simulink model "VD_correct"  (R2023b)
settings: Solver=ode15s  StartTime=0.0  StopTime=10.0  RelTol=1e-3
libraries: simulink x1
settings Model: Creator=Supriya  LastModifiedBy=Supriya

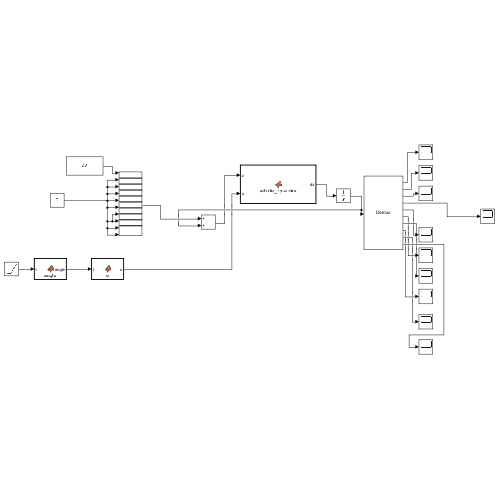
[thumbnail: Simulink's stored preview of the top-level diagram]
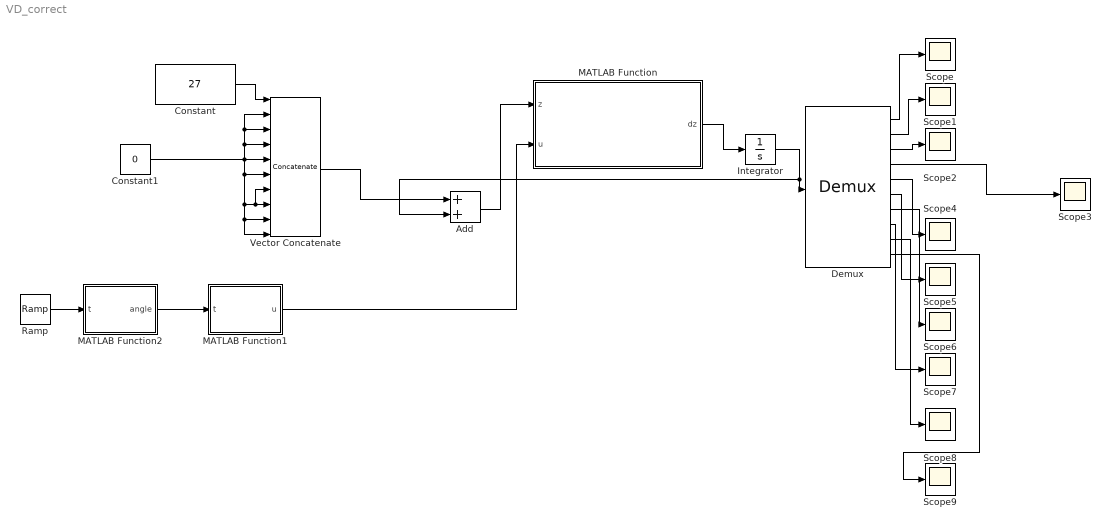
== system VD_correct ==
  Add : Sum
  Constant : Constant  Value=27
  Constant1 : Constant  Value=0
  Demux : Demux  Outputs=10
      settings: DisplayOption=none
  Integrator : Integrator
  MATLAB Function : MATLAB Function  TreatAsAtomicUnit=on
  MATLAB Function1 : MATLAB Function  TreatAsAtomicUnit=on
  MATLAB Function2 : MATLAB Function  TreatAsAtomicUnit=on
  Ramp : simulink/Sources/Ramp  slope=1  start=0  InitialOutput=0
  Scope{,1..9} (10 alike) : Scope
  Vector Concatenate : Concatenate  NumInputs=10
  wires:
  MATLAB Function/1(dz) -> Integrator/1
  Constant1/1 -> Vector Concatenate/3, Vector Concatenate/2, Vector Concatenate/4, Vector Concatenate/10, Vector Concatenate/9, Vector Concatenate/7, Vector Concatenate/8, Vector Concatenate/6, Vector Concatenate/5
  Vector Concatenate/1 -> Add/1
  Constant/1 -> Vector Concatenate/1
  Integrator/1 -> Demux/1, Add/2
  Demux/1 -> Scope/1
  Demux/2 -> Scope1/1
  Demux/3 -> Scope2/1
  Demux/4 -> Scope3/1
  Demux/5 -> Scope4/1
  Demux/6 -> Scope5/1
  Demux/7 -> Scope6/1
  Demux/8 -> Scope7/1
  MATLAB Function2/1(angle) -> MATLAB Function1/1(t)
  MATLAB Function1/1(u) -> MATLAB Function/2(u)
  Ramp/1 -> MATLAB Function2/1(t)
  Add/1 -> MATLAB Function/1(z)
  Demux/9 -> Scope8/1
  Demux/10 -> Scope9/1

== matlab function VD_correct/MATLAB Function1 ==
  data: t input; u output
function u = u(t)
    u=[1; 0; angle(t);];
end

== matlab function VD_correct/MATLAB Function ==
  data: dz output; z input; u input
function dz = vehicle_dynamics(z, u)
    % abc = Forces
    % dt;
    %tic;    
    accel = u(1);
    deccel = u(2);
    delta = u(3);
    function params = system_parameters();
        params.m = 2000; %kg
        params.rho = 1.225; %kg /m3
        params.C_d = 0.4; %
        params.Af = 1.6; %frontal area of vehicle 
        params.V_wind = 10 ;  %m/s
        params.a = 1.1;         %front_axel - CG
        params.b = 1.2;         % rear axel - CG
        params.l =  1.1 + 1.2;  %%m length of wheel base
        params.tf =  1.58; % track idth of wheel base 
        params.tr = 1.58; % track width of rear wheel base
        params.w = 1.58; % vehicle width
        params.Izz_v = 2000 * ((1.1+1.2)^2 + (1.58)^2) / 12;  %vehicle intertia 
        params.max_torque = 450; %Nm
        params.max_power =  225* 10^3;
        params.C_x = 50000 ;     %N
        params.C_y = 40000 ;  %N/Radlateral coefficient of stiffness
        params.R_f = 0.334; % m 
        params.R_r = 0.334; % m
        params.tire_m_f = 12; %mass in Kg
        params.tire_m_r = 12; %mass in Kg
        params.Iyy_w_f = 0.5 * 12 * 0.334; 
        params.Iyy_w_r = 0.5 * 12 * 0.334;
        % params.slip_max = (params.max_torque * accel / (params.R_f *2 * params.C_x));
        params.slip_min = -0.1;
        params.no_drive_wheels = 2;
        params.g = 9.8; %m/s2
        params.h = 0.25; %m
    end
    function slip_angles =  calculate_slip_angles(params,z, delta);


        Vx = z(1);
        Vy = z(2);
        r =  z(3);
        
        % term_a = atan2( (Vy + params.a * r ), ( Vx - (r * params.tf /2)) );
        % term_b = atan2( (Vy + params.a * r ), ( Vx + (r * params.tf /2)) );
        % term_c = atan2( (Vy - params.b * r ), ( Vx - (r * params.tr /2)) );
        % term_d = atan2( (Vy - params.b * r ), ( Vx + (r * params.tf /2)) );
    
        term_a = atan2( (Vy + params.a * r ),  Vx  );
        term_b = atan2( (Vy + params.a * r ),  Vx );
        term_c = atan2( (Vy - params.b * r ),  Vx );
        term_d = atan2( (Vy - params.b * r ),  Vx  );
    
        alpha_fl =  delta - term_a; if isnan(term_a ), alpha_fl = 0; end 
        alpha_fr =  delta - term_b; if isnan(term_b), alpha_fr = 0; end 
        alpha_rl = -term_c; if isnan(term_c), alpha_rl = 0; end
        alpha_rr = -term_d; if isnan(term_d), alpha_rr = 0; end
        
        slip_angles = -1 * [alpha_fl ; alpha_fr; alpha_rl; alpha_rr ];

    end
    params = system_parameters();
    function slips = caculate_slip(params, z ,deccel)
        %wheel longitudinal velocity and angular rate
        Vx = z(1);
        r = z(3);
        %%calculate linear velocities of each wheel 
           V_fl = Vx - (r * params.tf /2);
           V_fr = Vx + (r * params.tf /2);
           V_rl = Vx - (r * params.tr /2);
           V_rr = Vx + (r * params.tr /2);
           w_fl = z(7);
           w_fr = z(8);
           w_rl = z(9);
           w_rr = z(10); 
          
          if deccel > 0
            D1 = V_fl; 
            D2 = V_fr;
            D3 = V_rl;
            D4 = V_rr;
          else
            D1 = params.R_f * w_fl;
            D2 = params.R_f * w_fr;
            D3 = params.R_r * w_rl;
            D4 = params.R_r * w_rr;
          end
        
         S_fl = (params.R_f * w_fl - V_fl )/ D1; if (w_fl ==0), S_fl = 0; end 
         S_fr = (params.R_f * w_fr - V_fr) / D2; if (w_fr ==0), S_fr = 0; end
         S_rl = (params.R_r * w_rl - V_rl) / D3; if (w_rl ==0), S_rl = 0; end
         S_rr = (params.R_r * w_rr - V_rr )/ D4; if (w_rr ==0), S_rr = 0; end
      
         slips = [S_fl; S_fr; S_rl; S_rr];

    end
    function f_vector = tire_forces(params, z, delta, ax, ay, deccel)
        %% vehicle forces <- tire forces <- slip and normal forces <- angular wheel and 
        %% linear axel velocity <- T_inout & T_load <- accel, deccel   
           
    %%%%%%%%%%%%%%%%%%%%%%%%%%%%%%%%%%%%%%%%
    % Weight distribution (assuming 50-50 split)
    weight_front = 0.5;  % Percentage of weight on front axle
    weight_rear = 1 - weight_front;  % Percentage on rear axle
    
    % Static normal forces without acceleration
    F_drag =air_drag_force(params, z);
    load_transfer_longitudinal = (params.m * ax * params.h) / params.l;
    Fz_front = ((weight_front * params.m * params.g * params.b) - load_transfer_longitudinal - F_drag * params.h) / params.l;   % Force on each front tire
    Fz_rear = ((weight_rear * params.m * params.g * params.a) + load_transfer_longitudinal + F_drag * params.h) / params.l;     % Force on each rear tire
    
    
    
    % Load transfer due to lateral acceleration (cornering)
    %load_transfer_lateral = (params.m * ay * params.h) / params.tf;
    
    % Normal forces on each tire
    Fz_fl = Fz_front/2 ;  % Front-left tire
    Fz_fr = Fz_front/2;  % Front-right tire
    Fz_rl = Fz_rear/2;   % Rear-left tire
    Fz_rr = Fz_rear/2;   % Rear-right tire
    
    
    F_z = [Fz_fl, Fz_fr, Fz_rl, Fz_rr]';
    %%%%%%%%%%%%%%%%%%%%%%%%%%%%%%%%%%%%%%%%%%%
    
        
        Slips = caculate_slip(params, z,deccel);
    
        F_x=fricx(Slips ,F_z); %% Fx = [Fflx Ffrx Frlx Frrx]T - longitudinal forces are calulated using slip ratio -> 
                                                            % friction is calculated from that
        
        alpha = calculate_slip_angles(params,z, delta );                                                    % fx = f * fz
        F_y=fricy(alpha,F_z); %%  Fy = [Ffly Ffry Frly Frry]T - lateral forces calculation using similar logic
        
        
        f_vector = [F_x' , F_y'];
    end

 
    Vx =  z(1);
    Vy = z(2);
    r  = z(3);
    x  = z(4);
    y  = z(5);
    psi= z(6);
    ax = -z(2) * r;
    ay = z(1) * r;

    %%input torue to each wheel 
    tau_in = cal_wheel_torque_in(params, accel, deccel);
    tau_in_fl = tau_in(1);
    tau_in_fr = tau_in(2);
    tau_in_rl = tau_in(3);
    tau_in_rr = tau_in(4);
    
    %% calculate forces
    t_forces = tire_forces(params, z, delta, ax, ay, deccel); %8 * 1 vector
    [Fx_sum, Fy_f, Fy_r, Fy_del] = vehicle_forces(params, z, t_forces, delta);
        
    Vx_dt = Vy * r + (Fx_sum / params.m);
    Vy_dt = -Vx * r + ((Fy_f+ Fy_r) / params.m);

    t_forces = tire_forces(params, z, delta, Vx_dt, Vy_dt,deccel); %8 * 1 vector
    [Fx_sum, Fy_f, Fy_r, Fy_del] = vehicle_forces(params, z, t_forces, delta);


    Vx_dt = Vy * r + (Fx_sum / params.m);
    Vy_dt = -Vx * r + ((Fy_f+ Fy_r) / params.m);
    r_dt =  (params.a * Fy_f - params.b *Fy_r + Fy_del) / params.Izz_v;

    x_dt = Vx * cos(psi) - Vy * sin(psi);
    y_dt = Vx * sin(psi) + Vy * cos(psi);
    psi_dt  = r;    

    %set tire forces 
    Fx_fl = t_forces(1);
    Fx_fr = t_forces(2);
    Fx_rl = t_forces(3);
    Fx_rr = t_forces(4); 

    %wheel velocities 
    w_fl_dt = (tau_in_fl - Fx_fl * params.R_f) / params.Iyy_w_f;
    w_fr_dt = (tau_in_fr - Fx_fr * params.R_f) / params.Iyy_w_f;
    w_rl_dt = (tau_in_rl - Fx_rl * params.R_r) / params.Iyy_w_r;
    w_rr_dt = (tau_in_rr - Fx_rr * params.R_r) / params.Iyy_w_r;

    omega_fl_dt = w_fl_dt;
    omega_fr_dt = w_fr_dt;
    omega_rl_dt = w_rl_dt;
    omega_rr_dt = w_rr_dt;
    %tp = toc;
    dz = [Vx_dt; Vy_dt; r_dt; x_dt; y_dt; psi_dt; omega_fl_dt; omega_fr_dt; omega_rl_dt; omega_rr_dt];

    % ax = (Vx_dt -ax)/dt;
    % ay = (Vy_dt - ay)/dt;
    % 
    %dz = [Vx_dt; Vy_dt; r_dt; x_dt; y_dt; psi_dt; omega_fl_dt; omega_fr_dt; omega_rl_dt; omega_rr_dt; ax; ay];


end

== matlab function VD_correct/MATLAB Function2 ==
  data: t input; angle output
function angle = angle(t)
    % if t<1
    %     angle_steer = 0;%(pi/180) * sin(2*pi*0.1*t);
    % elseif 2>=t>=1
    %     angle_steer = 0.5*(pi/180)*t;
    % else
    %     angle_steer=2*0.5*(pi/180);
    % end
    angle_steer = (pi/180) * sin(2*pi*0.1*t);
    angle=angle_steer;
end
